simulink library "simlib_vpc_coremath"  (R2022a)
settings: Solver=VariableStepAuto  StartTime=0.0  StopTime=10.0  RelTol=1e-3
libraries: $bdroot x2
settings Model: Creator=marco  LastModifiedBy=marco
settings SolverCC: AlgebraicLoopSolver=TrustRegion
settings DebuggingCC: UnconnectedInputMsg=warning  UnconnectedOutputMsg=warning  UnconnectedLineMsg=warning  SFMachineParentedDataDiag=warning
settings RTWCC: DLArmComputeVersion=19.05

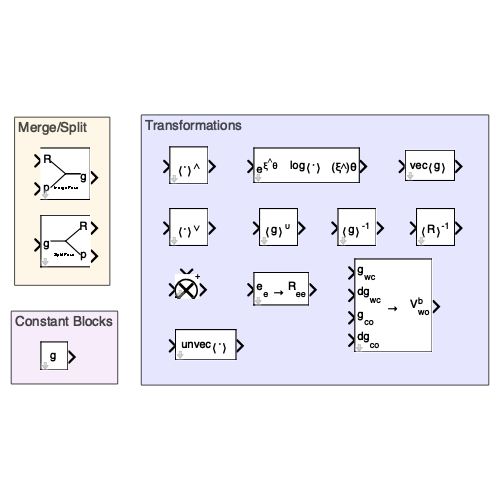
[thumbnail: Simulink's stored preview of the top-level diagram]
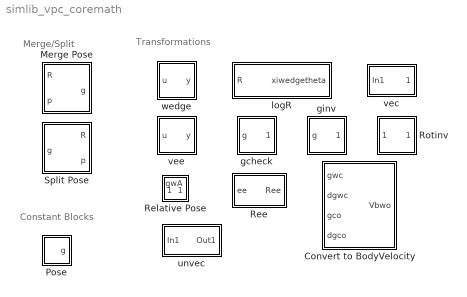
== system simlib_vpc_coremath ==
  note: Constant Blocks
  note: Transformations
  note: Merge/Split
  Convert to BodyVelocity : Subsystem  TreatAsAtomicUnit=on  mask(Convert to Body Velocity [V1]){}
      mask help:
      | Returns the body velocity V^b_{wo}.
      | Uses the inverse relation
      | V^b_{wo} = g_{wo}^{-1}\dot{g}_{wo}
      | with
      | \dot{g}_{wo} = \dot{g}_{wc}g_{co} + g_{wc}\dot{g}_{co}
      settings: MinAlgLoopOccurrences=on
      mask Help:
      | Refer to:
      | M. Omainska, J. Yamauchi, T. Beckers, T. Hatanaka, S. Hirche, and M.Fujita, <i>Gaussian Process Based Visual Pursuit Control with Unknown Target Motion Learning in Three Dimensions</i>, SICE Journal of Control, Measurement, and System Integration, Vol. 4, No. 1, pp. 001–009, January 2021.
      mask Display:
      | % Glitch in Matlab: If you define a line whose starting point and end point
      | % is equal, then the entire mask block is plotted in bold
      | plot([0,0],[0,0])
      | 
      | % Box
      | plot([0,1,1,0,0],[0,0,1,1,0])
      | 
      | % Write label
      | disp('\rightarrow','texmode','on')
      | 
      | % Label ports
      | port_label('input',1,'g_{wc}','texmode','on')
      | port_label('input',2,'dg_{wc}','texmode','on')
      | port_label('input',3,'g_{co}','texmode','on')
      | port_label('input',4,'dg_{co}','texmode','on')
      | port_label('output',1,'V^b_{wo}','texmode','on')
  Merge Pose : Subsystem  TreatAsAtomicUnit=on  mask(Merge pose [V1]){}
      mask help:
      | Forms pose as its homogeneous representation form:
      |
      | g = [R, p
      |         0, 1]
      |
      | The variables R and p denote the rotation matrix [size 3x3] and position vector [size 3], respectively.
      mask Help:
      | Refer to:
      | T. Hatanaka, N. Chopra, M. Fujita, and M. W. Spong, <i>Passivity-based Control and Estimation in Networked Robotics</i>, ser. Communications and Control Engineering. Springer, 2015.
      mask Display:
      | % Glitch in Matlab: If you define a line whose starting point and end point
      | % is equal, then the entire mask block is plotted in bold
      | plot([0.5,0.5],[0.5,0.5])
      | 
      | % "Fork"
      | plot([0.2,0.5,0.8],[0.75,0.5,0.5])
      | plot([0.2,0.5,0.8],[0.25,0.5,0.5])
      | plot([0,1,1,0],[0,0,1,1])
      | 
      | % Write label
      | text(0.3,0.3,'\fontsize{4}Merge Pose','texmode','on')
      | 
      | % Label ports
      | port_label('input',1,'R','texmode','on')
      | port_label('input',2,'p','texmode','on')
      | port_label('output',1,'g','texmode','on')
  Pose : Subsystem  TreatAsAtomicUnit=on  mask(Pose [V1]){R=[], p=[]}
      mask prompts: R "Rotation matrix R"; p "Position vector p"
      mask help:
      | Constant pose block.
      | Constructs a pose matrix from a rotation matrix and a position:
      |
      | g = [R, p
      |         0, 1]
      |
      | The variables R and p denote the rotation matrix [size 3x3] and position vector [size 3], respectively.
      mask init:
      | if isempty(R) || isscalar(R) && R == 0
      |     R = eye(3);
      | end
      | if isempty(p) || isscalar(p) && p == 0
      |     p = [0 0 0];
      | end
      | assert(all(size(R) == 3),'Invalid rotation matrix!');
      | assert(length(p(:)) == 3,'Invalid position vector!');
      | g_const = mergepose(R,p);
      mask Help:
      | Refer to:
      | T. Hatanaka, N. Chopra, M. Fujita, and M. W. Spong, <i>Passivity-based Control and Estimation in Networked Robotics</i>, ser. Communications and Control Engineering. Springer, 2015.
      mask Display:
      | % Glitch in Matlab: If you define a line whose starting point and end point
      | % is equal, then the entire mask block is plotted in bold
      | plot([0,0],[0,0])
      | 
      | % Box
      | plot([0,1,1,0,0],[0,0,1,1,0])
      | 
      | % Write label
      | blockpos = get_param(gcb,'Position');
      | x1 = blockpos(1); x2 = blockpos(3);
      | y1 = blockpos(2); y2 = blockpos(4);
      | if x2 - x1 >= 40 && y2 - y1 >= 40
      |     R = eval(get_param(gcb, 'R'));
      |     p = eval(get_param(gcb, 'p'));
      |     if isempty(R) || isscalar(R) && R == 0
      |         R = eye(3);
      |     end
      |     if isempty(p) || isscalar(p) && p == 0
      |         p = [0 0 0];
      |     end
      |     g = mergepose(R,p);
      |     %disp(strjoin(string(num2str(g,'% -.2g ')),'\n'));
      |     disp(string(num2str(g,'% -.2g ')));
      | else
      |     disp('g','texmode','on')
      | end
  Ree : Subsystem  TreatAsAtomicUnit=on  mask(Rotation Estimation Error [V1]){}
      mask help:
      | Returns the rotational error in the estimation.
      |
      | Under the assumption that the estimation error angle is bounded by |θ_ee| ≤ π/2, the estimation rotation error R = e^{xi^{∨}*θ_ee} can be calculated [2] by its vectorized skew-form skRv = sk(R)^{∨} as:
      | R = asin(||skRv||)/||skRv|| * skRv
      |
      | The input to this block can be either the estimation error ee [size 6], or directly the vee-transformed skew rotation error skRv [size 3].
      mask Help:
      | Refer to:
      | [1] T. Hatanaka, N. Chopra, M. Fujita, and M. W. Spong, <i>Passivity-based Control and Estimation in Networked Robotics</i>, ser. Communications and Control Engineering. Springer, 2015.
      | [2] T. Murao, H. Kawai, M. Fujita, <i>Predictive visual feedback control with eye-in/to-hand configuration via stabilizing receding horizon approach.</i> IFAC Proc Vol.2008;41(2):5341–5346.
      mask Display:
      | % Glitch in Matlab: If you define a line whose starting point and end point
      | % is equal, then the entire mask block is plotted in bold
      | plot([0,0],[0,0])
      | 
      | % Box
      | plot([0,1,1,0,0],[0,0,1,1,0])
      | 
      | % Write label
      | % disp('Rotation Estimation Error','texmode','on')
      | disp('\rightarrow ','texmode','on')
      | % disp('e^{\xi^{\wedge}\theta_{ee}}','texmode','on')
      | 
      | % Label ports
      | port_label('input',1,'e_e','texmode','on')
      | % port_label('output',1,'e^{\xi^{\wedge}\theta_{ee}}','texmode','on')
      | port_label('output',1,'R_{ee}','texmode','on')
  Relative Pose : Subsystem  TreatAsAtomicUnit=on  mask(Relative Pose Block [V1]){}
      mask help:
      | <!DOCTYPE html>
      | <html>
      | <body>
      |
      | <p>Simply returns the relative pose from frame A seen from frame B.</p>
      |
      | </body>
      | </html>
      settings: PortSchema="{\"entries\":[{\"content\":{\"sides\":[{\"content\":{\"connectorIds\":[\"In1\"]},\"type\":\"ConnectorPlacement.EquallySpacedRectSide\",\"uuid\":\"3d122c75-6063-48d0-bdc6-e48d95f4f0df\"},{\"content\":{\"connectorIds\":[\"Out1\"],\"side\":\"RIGHT\"},\"type\":\"ConnectorPlacement.EquallySpacedRectSide\",\"uuid\":\"6f2baba1-0bbd-4647-86ee-c97990dc6bd4\"},{\"content\":{\"connectorIds\":[\"In2\"],\"side\":\"TOP\"},\"type\":\"ConnectorPlacement.EquallySpacedRectSide\",\"uuid\":\"e6bc68d2-46ec-4597-a68e-7f59d26336ee\"},{\"content\":{\"connectorIds\":[],\"side\":\"HIDDEN\"},\"type\":\"ConnectorPlacement.EquallySpacedRectSide\",\"uuid\":\"d66c6085-c61f-489e-b38a-36804ae2ee0b\"}]},\"type\":\"ConnectorPlacement.EquallySpacedConnector\",\"uuid\":\"9cb4cf54-89e1-4d8f-a4cb-7cce930f6af0\"}],\"packageUris\":[\"http://schema.mathworks.com/mf0/Connector/R2020b\"],\"version\":\"1.0\"}"
      mask Help:
      | Refer to:
      | T. Hatanaka, N. Chopra, M. Fujita, and M. W. Spong, <i>Passivity-based Control and Estimation in Networked Robotics</i>, ser. Communications and Control Engineering. Springer, 2015.
      mask Display:
      | % Glitch in Matlab: If you define a line whose starting point and end point
      | % is equal, then the entire mask block is plotted in bold
      | % plot([0.5,0.5],[0.5,0.5])
      | 
      | % "x"
      | % xwidth = round(sqrt(0.5)/2,2);
      | % plot([0.5-xwidth, 0.5+xwidth],[0.5-xwidth, 0.5+xwidth])
      | % plot([0.5-xwidth, 0.5+xwidth],[0.5+xwidth, 0.5-xwidth])
      | 
      | % Draw circle
      | % r = 0.5;
      | % ang=round([0:0.3:2*pi, 2*pi],1);
      | % xp=r*cos(ang);
      | % yp=r*sin(ang);
      | % plot(0.5+xp,0.5+yp);
      | 
      | % Write label
      | text(0.02,0.1,'\fontsize{15}-','texmode','on')
      | % text(0.85,0.95,'\fontsize{10}+','texmode','on')
      | text(0.85,1,'\fontsize{8}+','texmode','on')
      | 
      | 
      | % Write label
      | % text(0.2,0.35,'\fontsize{15}-','texmode','on')
      | % text(0.55,0.75,'\fontsize{10}+','texmode','on')
      | 
      | % Write label
      | p=get_param(gcb,'Position');
      | size = min(p(3:4)-p(1:2));
      | scale = round(55*(size/46));
      | % disp('\fontsize{32}\otimes','texmode','on')
      | disp(['\fontsize{' char(num2str(scale)) '}\otimes'],'texmode','on')
  Rotinv : Subsystem  TreatAsAtomicUnit=on  mask(Invert rotation [V1]){}
      mask help:
      | <!DOCTYPE html>
      | <html>
      | <body>
      |
      | <p>Calculates inverse of rotation <i>R</i>.</p>
      |
      | </body>
      | </html>
      mask Help:
      | Refer to:
      | T. Hatanaka, N. Chopra, M. Fujita, and M. W. Spong, <i>Passivity-based Control and Estimation in Networked Robotics</i>, ser. Communications and Control Engineering. Springer, 2015.
      mask Display:
      | % Glitch in Matlab: If you define a line whose starting point and end point
      | % is equal, then the entire mask block is plotted in bold
      | plot([0,0],[0,0])
      | 
      | % Box
      | plot([0,1,1,0,0],[0,0,1,1,0])
      | 
      | % Write label
      | disp('\langleR\rangle^{-1}','texmode','on')
  Split Pose : Subsystem  TreatAsAtomicUnit=on  mask(Split pose [V1]){show_R=on, show_p=on}
      mask prompts: show_R "Rotation matrix R"; show_p "Position vector p"
      mask help:
      | Extracts Rotation matrix and Position vector from homogeneous representation matrix of pose [size 4x4]
      |
      | g = [R, p
      |         0, 1]
      |
      | The variables R and p denote the rotation matrix [size 3x3] and position vector [size 3], respectively.
      mask init:
      | port_number = 1;
      | 
      | % Show / Hide: R
      | if show_R % Show output
      |     block = find_system(gcb,'SearchDepth','1','LookUnderMasks','on',...
      |         'FollowLinks','on','Name','R_terminator');
      |     try delete_line(gcb,'Split Pose/1','R_terminator/1'); catch; end
      |     try delete_block(block); catch; end
      |     try add_block('built-in/Outport',[gcb,'/R'],'Port',num2str(port_number),'Position',[145 33 175 47]); catch; end
      |     try add_line(gcb,'Split Pose/1','R/1','autorouting','smart'); catch; end
      |     port_number = port_number+1;
      | else % Hide output
      |     block = find_system(gcb,'SearchDepth','1','LookUnderMasks','on',...
      |         'FollowLinks','on','Name','R');
      |     try delete_line(gcb,'Split Pose/1','R/1'); catch; end
      |     try delete_block(block); catch; end
      |     try add_block('built-in/Terminator',[gcb,'/R_terminator'],'Position',[145 33 175 47]); catch; end
      |     try add_line(gcb,'Split Pose/1','R_terminator/1','autorouting','smart'); catch; end
      | end
      | 
      | % Show / Hide: p
      | if show_p % Show output
      |     block = find_system(gcb,'SearchDepth','1','LookUnderMasks','on',...
      |         'FollowLinks','on','Name','p_terminator');
      |     try delete_line(gcb,'Split Pose/1','p_terminator/1'); catch; end
      |     try delete_block(block); catch; end
      |     try add_block('built-in/Outport',[gcb,'/p'],'Port',num2str(port_number),'Position',[145 63 175 77]); catch; end
      |     try add_line(gcb,'Split Pose/1','p/1','autorouting','smart'); catch; end
      |     port_number = port_number+1;
      | else % Hide output
      |     block = find_system(gcb,'SearchDepth','1','LookUnderMasks','on',...
      |         'FollowLinks','on','Name','p');
      |     try delete_line(gcb,'Split Pose/1','p/1'); catch; end
      |     try delete_block(block); catch; end
      |     try add_block('built-in/Terminator',[gcb,'/p_terminator'],'Position',[145 63 175 77]); catch; end
      |     try add_line(gcb,'Split Pose/1','p_terminator/1','autorouting','smart'); catch; end
      | end
      mask Help:
      | Refer to:
      | T. Hatanaka, N. Chopra, M. Fujita, and M. W. Spong, <i>Passivity-based Control and Estimation in Networked Robotics</i>, ser. Communications and Control Engineering. Springer, 2015.
      mask DialogControl ValueGroupVar Prompt: Show outputs
      mask Display:
      | % Glitch in Matlab: If you define a line whose starting point and end point
      | % is equal, then the entire mask block is plotted in bold
      | plot([0,0],[0,0])
      | 
      | % Box
      | plot([1,0,0,1],[0,0,1,1])
      | 
      | % "Fork"
      | plot([0.2,0.5],[0.5,0.5])
      | show_R = get_param(gcb,'show_R');
      | show_p = get_param(gcb,'show_p');
      | if strcmp(show_R,'on') && strcmp(show_p,'on')
      |     plot([0.5,0.8],[0.5,0.75])
      |     plot([0.5,0.8],[0.5,0.25])
      | elseif strcmp(show_R,'on') || strcmp(show_p,'on')
      |     plot([0.5,0.8],[0.5,0.5])
      | end
      | 
      | % Write label
      | text(0.3,0.3,'\fontsize{4}Split Pose','texmode','on')
      | 
      | % Label ports
      | outport = 1;
      | port_label('input',1,'g','texmode','on')
      | if strcmp(show_R,'on')
      |     port_label('output',outport,'R','texmode','on')
      |     outport = outport + 1;
      | end
      | if strcmp(show_p,'on')
      |     port_label('output',outport,'p','texmode','on')
      |     outport = outport + 1;
      | end
  gcheck : Subsystem  TreatAsAtomicUnit=on  mask(Check Transform [V1]){}
      mask help:
      | <!DOCTYPE html>
      | <html>
      | <body>
      |
      | <p>Transforms pose <i>g</i> into check-transform <i>g<sup>&cup;</sup></i></p>
      |
      | </body>
      | </html>
      mask Help:
      | Refer to:
      | M. Omainska, J. Yamauchi, T. Beckers, T. Hatanaka, S. Hirche, and M.Fujita, <i>Gaussian Process Based Visual Pursuit Control with Unknown Target Motion Learning in Three Dimensions</i>, SICE Journal of Control, Measurement, and System Integration, Vol. 4, No. 1, pp. 001–009, January 2021.
      mask Display:
      | % Glitch in Matlab: If you define a line whose starting point and end point
      | % is equal, then the entire mask block is plotted in bold
      | plot([0,0],[0,0])
      | 
      | % Box
      | plot([0,1,1,0,0],[0,0,1,1,0])
      | 
      | % "Sink"
      | % plot([0,0.5,1],[1,1,0.7])
      | % plot([0,0.5,1],[0,0,0.3])
      | 
      | % Write label
      | disp('\langleg\rangle^{\upsilon}','texmode','on')
  ginv : Subsystem  TreatAsAtomicUnit=on  mask(Invert pose [V1]){}
      mask help:
      | <!DOCTYPE html>
      | <html>
      | <body>
      |
      | <p>Calculates inverse of pose <i>g</i>.</p>
      |
      | </body>
      | </html>
      mask Help:
      | Refer to:
      | T. Hatanaka, N. Chopra, M. Fujita, and M. W. Spong, <i>Passivity-based Control and Estimation in Networked Robotics</i>, ser. Communications and Control Engineering. Springer, 2015.
      mask Display:
      | % Glitch in Matlab: If you define a line whose starting point and end point
      | % is equal, then the entire mask block is plotted in bold
      | plot([0,0],[0,0])
      | 
      | % Box
      | plot([0,1,1,0,0],[0,0,1,1,0])
      | 
      | % Write label
      | disp('\langleg\rangle^{-1}','texmode','on')
  logR : Subsystem  TreatAsAtomicUnit=on  mask(Inverse rotation exponential function [V1]){}
      mask help:
      | Returns the argument of the exponential rotation matrix exp{xi^{wedge}*theta}.
      | In other words, the matrix xi^{wedge}*theta is returned.
      mask Help:
      | Refer to:
      | T. Hatanaka, N. Chopra, M. Fujita, and M. W. Spong, <i>Passivity-based Control and Estimation in Networked Robotics</i>, ser. Communications and Control Engineering. Springer, 2015.
      mask Display:
      | % Glitch in Matlab: If you define a line whose starting point and end point
      | % is equal, then the entire mask block is plotted in bold
      | plot([0,0],[0,0])
      | 
      | % Box
      | plot([0,1,1,0,0],[0,0,1,1,0])
      | 
      | % Write label
      | disp('log\langle\cdot\rangle','texmode','on')
      | 
      | % Label ports
      | port_label('input',1,'e^{\xi^{\wedge}\theta}','texmode','on')
      | port_label('output',1,'(\xi^{\wedge})\theta','texmode','on')
  unvec : Subsystem  TreatAsAtomicUnit=on  mask(Vec Transform [V1]){}
      mask help:
      | <!DOCTYPE html>
      | <html>
      | <body>
      |
      | <p>Back-Transform of vec-transformed <i>vec(g)</i> into the matrix pose form <i>g</i>.</p>
      |
      | </body>
      | </html>
      mask Help:
      | Refer to:
      | T. Hatanaka, N. Chopra, M. Fujita, and M. W. Spong, <i>Passivity-based Control and Estimation in Networked Robotics</i>, ser. Communications and Control Engineering. Springer, 2015.
      mask Display:
      | % Glitch in Matlab: If you define a line whose starting point and end point
      | % is equal, then the entire mask block is plotted in bold
      | plot([0,0],[0,0])
      | 
      | % Box
      | plot([0,1,1,0,0],[0,0,1,1,0])
      | 
      | % Write label
      | disp('unvec\langle{\cdot}\rangle','texmode','on')
      | 
      | % Label ports
      | %port_label('input',1,'x','texmode','on')
      | %port_label('output',1,'g','texmode','on')
  vec : Subsystem  TreatAsAtomicUnit=on  mask(Vec Transform [V1]){}
      mask help:
      | <!DOCTYPE html>
      | <html>
      | <body>
      |
      | <p>Transforms pose <i>g</i> into vec-transform <i>vec(g)</i>.</p>
      |
      | </body>
      | </html>
      mask Help:
      | Refer to:
      | T. Hatanaka, N. Chopra, M. Fujita, and M. W. Spong, <i>Passivity-based Control and Estimation in Networked Robotics</i>, ser. Communications and Control Engineering. Springer, 2015.
      mask Display:
      | % Glitch in Matlab: If you define a line whose starting point and end point
      | % is equal, then the entire mask block is plotted in bold
      | plot([0,0],[0,0])
      | 
      | % Box
      | plot([0,1,1,0,0],[0,0,1,1,0])
      | 
      | % Write label
      | disp('vec\langleg\rangle','texmode','on')
  vee : Subsystem  TreatAsAtomicUnit=on  mask(Vee Transform [V1]){}
      mask help:
      | <!DOCTYPE html>
      | <html>
      | <body>
      |
      | <p>Vee-transform of input <i>u</i> into <i>u<sup>&or;</sup></i></p>
      |
      | </body>
      | </html>
      mask Help:
      | Refer to:
      | T. Hatanaka, N. Chopra, M. Fujita, and M. W. Spong, <i>Passivity-based Control and Estimation in Networked Robotics</i>, ser. Communications and Control Engineering. Springer, 2015.
      mask Display:
      | % Glitch in Matlab: If you define a line whose starting point and end point
      | % is equal, then the entire mask block is plotted in bold
      | plot([0,0],[0,0])
      | 
      | % Box
      | plot([0,1,1,0,0],[0,0,1,1,0])
      | 
      | % Write label
      | disp('\langle\cdot\rangle^{\vee}','texmode','on')
  wedge : Subsystem  TreatAsAtomicUnit=on  mask(Wedge Transform [V1]){}
      mask help:
      | <!DOCTYPE html>
      | <html>
      | <body>
      |
      | <p>Wedge-transform of input <i>u</i> into <i>u<sup>&and;</sup></i></p>
      |
      | </body>
      | </html>
      mask Help:
      | Refer to:
      | T. Hatanaka, N. Chopra, M. Fujita, and M. W. Spong, <i>Passivity-based Control and Estimation in Networked Robotics</i>, ser. Communications and Control Engineering. Springer, 2015.
      mask Display:
      | % Glitch in Matlab: If you define a line whose starting point and end point
      | % is equal, then the entire mask block is plotted in bold
      | plot([0,0],[0,0])
      | 
      | % Box
      | plot([0,1,1,0,0],[0,0,1,1,0])
      | 
      | % Write label
      | disp('\langle\cdot\rangle^{\wedge}','texmode','on')

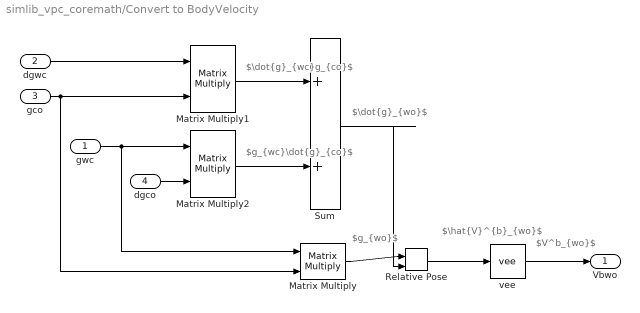
== system simlib_vpc_coremath/Convert to BodyVelocity ==
  note: $g_{wo}$
  note: $\dot{g}_{wc}g_{co}$
  note: $g_{wc}\dot{g}_{co}$
  note: $\dot{g}_{wo}$
  note: $\hat{V}^{b}_{wo}$
  note: $V^b_{wo}$
  gwc : Inport
  dgwc : Inport  Port=2
  gco : Inport  Port=3
  dgco : Inport  Port=4
  Matrix Multiply : Product  Multiplication=Matrix(*)
  Matrix Multiply1 : Product  Multiplication=Matrix(*)
  Matrix Multiply2 : Product  Multiplication=Matrix(*)
  Relative Pose : $bdroot/Relative Pose
  Sum : Sum
  vee : $bdroot/vee
  Vbwo : Outport
  wires:
  gco/1 -> Matrix Multiply/2, Matrix Multiply1/2
  gwc/1 -> Matrix Multiply/1, Matrix Multiply2/1
  Matrix Multiply/1 -> Relative Pose/1
  dgwc/1 -> Matrix Multiply1/1
  dgco/1 -> Matrix Multiply2/2
  Matrix Multiply1/1 -> Sum/1
  Matrix Multiply2/1 -> Sum/2
  Sum/1 -> Relative Pose/2
  Relative Pose/1 -> vee/1
  vee/1 -> Vbwo/1

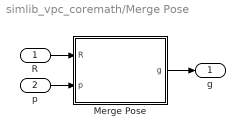
== system simlib_vpc_coremath/Merge Pose ==
  R : Inport
  p : Inport  Port=2
  Merge Pose : MATLAB Function  TreatAsAtomicUnit=on
  g : Outport
  wires:
  R/1 -> Merge Pose/1(R)
  Merge Pose/1(g) -> g/1
  p/1 -> Merge Pose/2(p)

== system simlib_vpc_coremath/Pose ==
  pose : Constant  Value=g_const
  g : Outport
  wires:
  pose/1 -> g/1

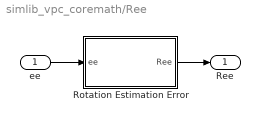
== system simlib_vpc_coremath/Ree ==
  ee : Inport
  Rotation Estimation Error : MATLAB Function  TreatAsAtomicUnit=on
  Ree : Outport
  wires:
  ee/1 -> Rotation Estimation Error/1(ee)
  Rotation Estimation Error/1(Ree) -> Ree/1

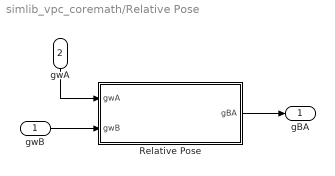
== system simlib_vpc_coremath/Relative Pose ==
  gwB : Inport
  gwA : Inport  Port=2
  Relative Pose : MATLAB Function  TreatAsAtomicUnit=on
  gBA : Outport
  wires:
  gwB/1 -> Relative Pose/2(gwB)
  Relative Pose/1(gBA) -> gBA/1
  gwA/1 -> Relative Pose/1(gwA)

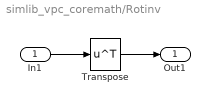
== system simlib_vpc_coremath/Rotinv ==
  In1 : Inport
  Transpose : Math  Operator=transpose  OutputSignalType=real
  Out1 : Outport
  wires:
  In1/1 -> Transpose/1
  Transpose/1 -> Out1/1

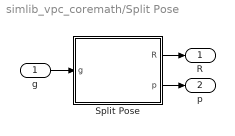
== system simlib_vpc_coremath/Split Pose ==
  g : Inport
  Split Pose : MATLAB Function  TreatAsAtomicUnit=on
  R : Outport
  p : Outport  Port=2
  wires:
  Split Pose/2(p) -> p/1
  g/1 -> Split Pose/1(g)
  Split Pose/1(R) -> R/1

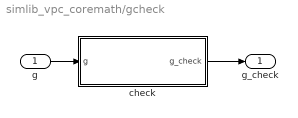
== system simlib_vpc_coremath/gcheck ==
  g : Inport
  check : MATLAB Function  TreatAsAtomicUnit=on
  g_check : Outport
  wires:
  g/1 -> check/1(g)
  check/1(g_check) -> g_check/1

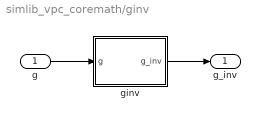
== system simlib_vpc_coremath/ginv ==
  g : Inport
  ginv : MATLAB Function  TreatAsAtomicUnit=on
  g_inv : Outport
  wires:
  g/1 -> ginv/1(g)
  ginv/1(g_inv) -> g_inv/1

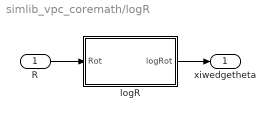
== system simlib_vpc_coremath/logR ==
  R : Inport
  logR : MATLAB Function  TreatAsAtomicUnit=on
  xiwedgetheta : Outport
  wires:
  R/1 -> logR/1(Rot)
  logR/1(logRot) -> xiwedgetheta/1

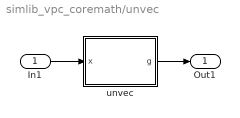
== system simlib_vpc_coremath/unvec ==
  In1 : Inport
  unvec : MATLAB Function  TreatAsAtomicUnit=on
  Out1 : Outport
  wires:
  In1/1 -> unvec/1(x)
  unvec/1(g) -> Out1/1

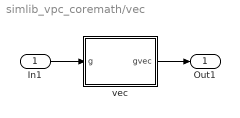
== system simlib_vpc_coremath/vec ==
  In1 : Inport
  vec : MATLAB Function  TreatAsAtomicUnit=on
  Out1 : Outport
  wires:
  In1/1 -> vec/1(g)
  vec/1(gvec) -> Out1/1

== system simlib_vpc_coremath/vee ==
  u : Inport
  vee : MATLAB Function  TreatAsAtomicUnit=on
  y : Outport
  wires:
  u/1 -> vee/1(u)
  vee/1(y) -> y/1

== system simlib_vpc_coremath/wedge ==
  u : Inport
  wedge : MATLAB Function  TreatAsAtomicUnit=on
  y : Outport
  wires:
  u/1 -> wedge/1(u)
  wedge/1(y) -> y/1

== matlab function simlib_vpc_coremath/Merge Pose/Merge Pose ==
  data R settings: description=Rotation matrix
  data g settings: description=|
      | Homogeneous representation of pose
      | 
      | g = [R, p
      |         0, 1]
  data p settings: description=Position vector
  data: R input size=[3,3]; g output size=[4,4]; p input size=3
function g = slx_mergepose(R,p) %#codegen
% Function Wrapper
%
% Editor:
%   OMAINSKA Marco - Doctoral Student, Cybernetics
%       <marcoomainska@g.ecc.u-tokyo.ac.jp>
% Review:
%   YAMAUCHI Junya - Assistant Professor
%       <junya_yamauchi@ipc.i.u-tokyo.ac.jp>
%
% Property of: Fujita-Yamauchi Lab, University of Tokyo, 2021
% e-mail: marcoomainska@g.ecc.u-tokyo.ac.jp
% Website: https://www.scl.ipc.i.u-tokyo.ac.jp
% March 2021, Last modified: 2021-MAR-08
%
%------------- BEGIN CODE --------------

% "mergepose" is a MATLAB function on the MATLAB path
g = mergepose(R,p);

%-------------- END CODE ---------------
end

== matlab function simlib_vpc_coremath/gcheck/check ==
  data: g input size=[4,4]; g_check output size=6
function g_check = slx_check(g) %#codegen
% Function Wrapper
%
% Editor:
%   OMAINSKA Marco - Doctoral Student, Cybernetics
%       <marcoomainska@g.ecc.u-tokyo.ac.jp>
% Review:
%   YAMAUCHI Junya - Assistant Professor
%       <junya_yamauchi@ipc.i.u-tokyo.ac.jp>
%
% Property of: Fujita Lab, University of Tokyo, 2021
% e-mail: marcoomainska@g.ecc.u-tokyo.ac.jp
% Website: https://www.scl.ipc.i.u-tokyo.ac.jp
% March 2021, Last modified: 2021-MAR-08
%
%------------- BEGIN CODE --------------

% "check" is a MATLAB function on the MATLAB path
g_check = check(g)';

%-------------- END CODE ---------------
end

== matlab function simlib_vpc_coremath/vee/vee ==
  data: u input; y output
function y = slx_vee(u) %#codegen
% Function Wrapper
%
% Editor:
%   OMAINSKA Marco - Doctoral Student, Cybernetics
%       <marcoomainska@g.ecc.u-tokyo.ac.jp>
% Review:
%   YAMAUCHI Junya - Assistant Professor
%       <junya_yamauchi@ipc.i.u-tokyo.ac.jp>
%
% Property of: Fujita-Yamauchi Lab, University of Tokyo, 2020
% e-mail: marcoomainska@g.ecc.u-tokyo.ac.jp
% Website: https://www.scl.ipc.i.u-tokyo.ac.jp
% March 2021, Last modified: 2021-MAR-08
%
%------------- BEGIN CODE --------------

% "vee" is a MATLAB function on the MATLAB path
y = vee(u);

%-------------- END CODE ---------------
end

== matlab function simlib_vpc_coremath/wedge/wedge ==
  data: u input; y output
function y = slx_wedge(u) %#codegen
% Function Wrapper
%
% Editor:
%   OMAINSKA Marco - Doctoral Student, Cybernetics
%       <marcoomainska@g.ecc.u-tokyo.ac.jp>
% Review:
%   YAMAUCHI Junya - Assistant Professor
%       <junya_yamauchi@ipc.i.u-tokyo.ac.jp>
%
% Property of: Fujita Lab, University of Tokyo, 2021
% e-mail: marcoomainska@g.ecc.u-tokyo.ac.jp
% Website: https://www.scl.ipc.i.u-tokyo.ac.jp
% March 2021, Last modified: 2021-MAR-08
%
%------------- BEGIN CODE --------------

% "wedge" is a MATLAB function on the MATLAB path
y = wedge(u);

%-------------- END CODE ---------------
end

== matlab function simlib_vpc_coremath/logR/logR ==
  data: Rot input size=[3,3]; logRot output size=[3,3]
function logRot = slx_logR(Rot) %#codegen
% Function Wrapper
%
% Editor:
%   OMAINSKA Marco - Doctoral Student, Cybernetics
%       <marcoomainska@g.ecc.u-tokyo.ac.jp>
% Review:
%   YAMAUCHI Junya - Assistant Professor
%       <junya_yamauchi@ipc.i.u-tokyo.ac.jp>
%
% Property of: Fujita Lab, University of Tokyo, 2021
% e-mail: marcoomainska@g.ecc.u-tokyo.ac.jp
% Website: https://www.scl.ipc.i.u-tokyo.ac.jp
% March 2021, Last modified: 2021-MAR-08
%
%------------- BEGIN CODE --------------

% "logR" is a MATLAB function on the MATLAB path
logRot = logR(Rot);

%-------------- END CODE ---------------
end

== matlab function simlib_vpc_coremath/vec/vec ==
  data: g input size=[4,4]; gvec output size=6
function gvec = slx_vec(g) %#codegen
% Function Wrapper
%
% Editor:
%   OMAINSKA Marco - Doctoral Student, Cybernetics
%       <marcoomainska@g.ecc.u-tokyo.ac.jp>
% Review:
%   YAMAUCHI Junya - Assistant Professor
%       <junya_yamauchi@ipc.i.u-tokyo.ac.jp>
%
% Property of: Fujita Lab, University of Tokyo, 2021
% e-mail: marcoomainska@g.ecc.u-tokyo.ac.jp
% Website: https://www.scl.ipc.i.u-tokyo.ac.jp
% March 2021, Last modified: 2021-MAR-09
%
%------------- BEGIN CODE --------------

% "vec" is a MATLAB function on the MATLAB path
gvec = vec(g);

%-------------- END CODE ---------------
end

== matlab function simlib_vpc_coremath/Relative Pose/Relative Pose ==
  data: gwA input size=[4,4]; gwB input size=[4,4]; gBA output size=[4,4]
function gBA = slx_relativePose(gwA, gwB) %#codegen
% Function Wrapper
%
% Editor:
%   OMAINSKA Marco - Doctoral Student, Cybernetics
%       <marcoomainska@g.ecc.u-tokyo.ac.jp>
% Review:
%   YAMAUCHI Junya - Assistant Professor
%       <junya_yamauchi@ipc.i.u-tokyo.ac.jp>
%
% Property of: Fujita-Yamauchi Lab, University of Tokyo, 2021
% e-mail: marcoomainska@g.ecc.u-tokyo.ac.jp
% Website: https://www.scl.ipc.i.u-tokyo.ac.jp
% March 2021, Last modified: 2021-MAR-08
%
%------------- BEGIN CODE --------------

% "relativePose" is a MATLAB function on the MATLAB path
gBA = relativePose(gwA, gwB);

%-------------- END CODE ---------------
end

== matlab function simlib_vpc_coremath/ginv/ginv ==
  data: g input size=[4,4]; g_inv output size=[4,4]
function g_inv = slx_ginv(g) %#codegen
% Function Wrapper
%
% Editor:
%   OMAINSKA Marco - Doctoral Student, Cybernetics
%       <marcoomainska@g.ecc.u-tokyo.ac.jp>
% Review:
%   YAMAUCHI Junya - Assistant Professor
%       <junya_yamauchi@ipc.i.u-tokyo.ac.jp>
%
% Property of: Fujita-Yamauchi Lab, University of Tokyo, 2021
% e-mail: marcoomainska@g.ecc.u-tokyo.ac.jp
% Website: https://www.scl.ipc.i.u-tokyo.ac.jp
% March 2021, Last modified: 2021-MAR-08
%
%------------- BEGIN CODE --------------

% "ginv" is a MATLAB function on the MATLAB path
g_inv = ginv(g);

%------------- END CODE --------------
end

== matlab function simlib_vpc_coremath/Ree/Rotation Estimation Error ==
  data: ee input; Ree output size=[3,3]
function Ree = slx_Ree(ee) %#codegen
% Function Wrapper
%
% Editor:
%   OMAINSKA Marco - Doctoral Student, Cybernetics
%       <marcoomainska@g.ecc.u-tokyo.ac.jp>
% Review:
%   YAMAUCHI Junya - Assistant Professor
%       <junya_yamauchi@ipc.i.u-tokyo.ac.jp>
%
% Property of: Fujita Lab, University of Tokyo, 2021
% e-mail: marcoomainska@g.ecc.u-tokyo.ac.jp
% Website: https://www.scl.ipc.i.u-tokyo.ac.jp
% March 2021, Last modified: 2021-MAR-08
%
%------------- BEGIN CODE --------------

% "Rotee" is a MATLAB function on the MATLAB path
Ree = Rotee(ee);

%-------------- END CODE ---------------
end

== matlab function simlib_vpc_coremath/unvec/unvec ==
  data: x input size=6; g output size=[4,4]
function g = slx_unvec(x) %#codegen
% Function Wrapper
%
% Editor:
%   OMAINSKA Marco - Doctoral Student, Cybernetics
%       <marcoomainska@g.ecc.u-tokyo.ac.jp>
% Review:
%   YAMAUCHI Junya - Assistant Professor
%       <junya_yamauchi@ipc.i.u-tokyo.ac.jp>
%
% Property of: Fujita Lab, University of Tokyo, 2022
% e-mail: marcoomainska@g.ecc.u-tokyo.ac.jp
% Website: https://www.scl.ipc.i.u-tokyo.ac.jp
% April 2022
%
%------------- BEGIN CODE --------------

% "unvec" is a MATLAB function on the MATLAB path
g = unvec(x);

%-------------- END CODE ---------------
end

== matlab function simlib_vpc_coremath/Split Pose/Split Pose ==
  data g settings: description=|
      | Homogeneous representation of pose
      | 
      | g = [R, p
      |         0, 1]
  data R settings: description=Rotation matrix R
  data p settings: description=Position vector p
  data: g input size=[4,4]; R output size=[3,3]; p output size=3
function [R,p] = slx_splitpose(g) %#codegen
% Function Wrapper
%
% Editor:
%   OMAINSKA Marco - Doctoral Student, Cybernetics
%       <marcoomainska@g.ecc.u-tokyo.ac.jp>
% Review:
%   YAMAUCHI Junya - Assistant Professor
%       <junya_yamauchi@ipc.i.u-tokyo.ac.jp>
%
% Property of: Fujita-Yamauchi Lab, University of Tokyo, 2021
% e-mail: marcoomainska@g.ecc.u-tokyo.ac.jp
% Website: https://www.scl.ipc.i.u-tokyo.ac.jp
% March 2021, Last modified: 2021-MAR-08
%
%------------- BEGIN CODE --------------

% "splitpose" is a MATLAB function on the MATLAB path
[R,p] = splitpose(g);

%-------------- END CODE ---------------
end
